simulink model "L_inf_allocation_test"  (R2018b)
settings: Solver=VariableStepAuto  StartTime=0.0  StopTime=10.0  RelTol=1e-3
undefined symbols (not defined in the file): fswParams
libraries: L_inf_allocation_lib x1
settings Model: Creator=taylorreynolds  LastModifiedBy=Taylor

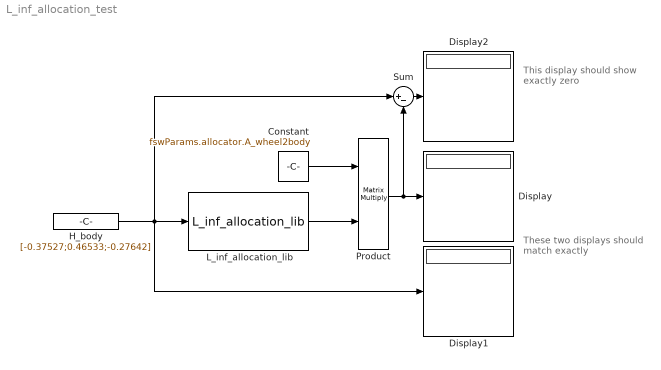
== system L_inf_allocation_test ==
  note: These two displays
      | should match exactly
  note: This display should
      | show exactly zero
  Constant : Constant  Value=fswParams.allocator.A_wheel2body
  Display : Display
  Display1 : Display
  Display2 : Display
  H_body : Constant  Value=[-0.37527;0.46533;-0.27642]
  L_inf_allocation_lib : L_inf_allocation_lib/L_inf_allocation_lib  SystemSampleTime=-1
  Product : Product  Multiplication=Matrix(*)
  Sum : Sum  Inputs=|+-
  wires:
  H_body/1 -> Sum/1, L_inf_allocation_lib/1, Display1/1
  L_inf_allocation_lib/1 -> Product/2
  Constant/1 -> Product/1
  Product/1 -> Sum/2, Display/1
  Sum/1 -> Display2/1
